simulink model "um_simulation"  (Simulink 8.2)
settings: Solver=ode8  StartTime=0.0  StopTime=120  RelTol=1e-3
settings Model: Creator=petter  LastModifiedBy=petter
settings DataIOCC: SaveOutput=off  SaveTime=off
settings OptimizationCC: ExpressionDepthLimit=128
settings DebuggingCC: MultiTaskDSMMsg=warning  MultiTaskCondExecSysMsg=none  FcnCallInpInsideContextMsg=EnableAllAsError
settings RTWCC: IncludeERTFirstTime=on
settings GRTTargetCC: CombineOutputUpdateFcns=on  GRTInterface=off

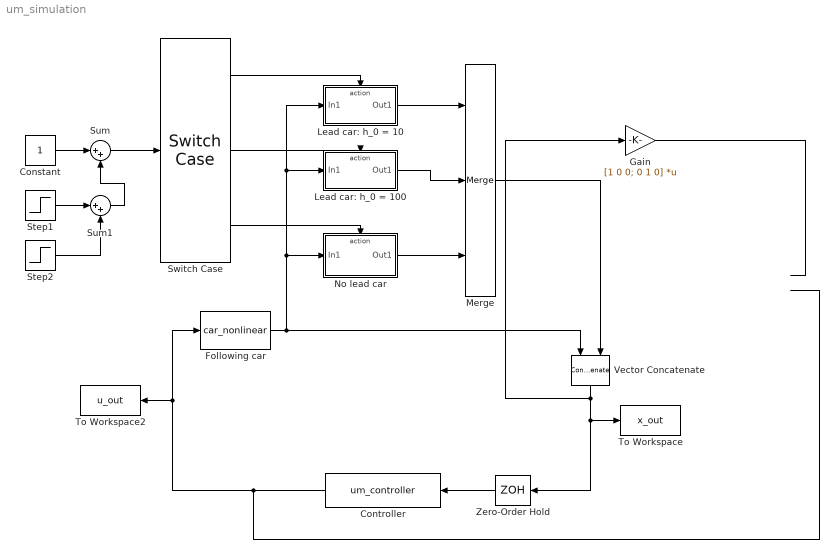
== system um_simulation ==
  Constant : Constant
  Controller : M-S-Function  FunctionName=um_controller
  Following car : M-S-Function  FunctionName=car_nonlinear
  Gain : Gain  Gain=[1 0 0; 0 1 0]  Multiplication=Matrix(K*u)
  "Lead car: h_0 = 10 " : Subsystem  TreatAsAtomicUnit=on
  Lead car: h_0 = 100 : Subsystem  TreatAsAtomicUnit=on
  Merge : Merge  Inputs=3
  No lead car : Subsystem  TreatAsAtomicUnit=on
  Step1 : Step  Time=60  After=-2  SampleTime=0
  Step2 : Step  Time=75  After=3  SampleTime=0
  Sum : Sum  Inputs=|++
  Sum1 : Sum  Inputs=|++
  Switch Case : SwitchCase  CaseConditions={1,2}
  To Workspace : ToWorkspace  VariableName=x_out  SampleTime=-1  SaveFormat=Structure With Time
  To Workspace2 : ToWorkspace  VariableName=u_out  SampleTime=-1  SaveFormat=Structure With Time
  Vector Concatenate : Concatenate
  Zero-Order Hold : ZeroOrderHold  SampleTime=0.02
  wires:
  Controller/1 -> Following car/1, To Workspace2/1
  Zero-Order Hold/1 -> Controller/1
  No lead car/1(Out1) -> Merge/3
  Merge/1 -> Vector Concatenate/2
  Vector Concatenate/1 -> Gain/1, To Workspace/1, Zero-Order Hold/1
  Step1/1 -> Sum1/1
  Constant/1 -> Sum/1
  "Lead car: h_0 = 10 "/1(Out1) -> Merge/1
  Switch Case/1 -> "Lead car: h_0 = 10 "/Action
  Following car/1 -> "Lead car: h_0 = 10 "/1(In1), Lead car: h_0 = 100/1(In1), No lead car/1(In1), Vector Concatenate/1
  Sum/1 -> Switch Case/1
  Sum1/1 -> Sum/2
  Step2/1 -> Sum1/2
  Switch Case/3 -> No lead car/Action
  Switch Case/2 -> Lead car: h_0 = 100/Action
  Lead car: h_0 = 100/1(Out1) -> Merge/2
  Gain/1 -> ?

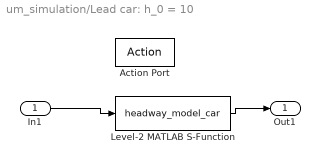
== system um_simulation/Lead car: h_0 = 10  ==
  In1 : Inport
  Action Port : ActionPort  InitializeStates=reset  ActionType=case
  Level-2 MATLAB S-Function : M-S-Function  FunctionName=headway_model_car  Parameters=200,10
  Out1 : Outport
  wires:
  In1/1 -> Level-2 MATLAB S-Function/1
  Level-2 MATLAB S-Function/1 -> Out1/1

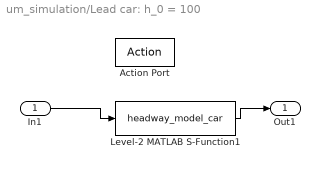
== system um_simulation/Lead car: h_0 = 100 ==
  In1 : Inport
  Action Port : ActionPort  InitializeStates=reset  ActionType=case
  Level-2 MATLAB S-Function1 : M-S-Function  FunctionName=headway_model_car  Parameters=120,12
  Out1 : Outport
  wires:
  In1/1 -> Level-2 MATLAB S-Function1/1
  Level-2 MATLAB S-Function1/1 -> Out1/1

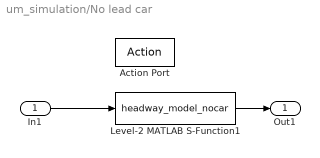
== system um_simulation/No lead car ==
  In1 : Inport
  Action Port : ActionPort  InitializeStates=reset  ActionType=default
  Level-2 MATLAB S-Function1 : M-S-Function  FunctionName=headway_model_nocar  Parameters=300.1
  Out1 : Outport
  wires:
  In1/1 -> Level-2 MATLAB S-Function1/1
  Level-2 MATLAB S-Function1/1 -> Out1/1
